simulink model "RADTRANS001"  (R2020b)
settings: Solver=VariableStepAuto  StartTime=0.0  StopTime=10.0  RelTol=1e-3
undefined symbols (not defined in the file): Line_110_C, Line_110_L, Line_110_R, Line_220_C, Line_220_L, Line_220_R, Line_35_C, Line_35_L, Line_35_R, Line_6_L, Line_6_R, Sys_f_Hz, Sys_V_net_kV, Tr_110_35_L_pu, Tr_110_35_R_pu, Tr_110_35_Sn_VA, Tr_110_35_V_HV_kV, Tr_110_35_V_LV_kV, Tr_110_6_L_pu, Tr_110_6_R_pu, Tr_110_6_Sn_VA, Tr_110_6_V_HV_kV, Tr_110_6_V_LV_kV, Tr_220_110_L_pu, Tr_220_110_R_pu, Tr_220_110_Sn_VA, Tr_220_110_V_HV_kV, Tr_220_110_V_LV_kV, Tr_35_04_L_pu, Tr_35_04_R_pu, Tr_35_04_Sn_VA, Tr_35_04_V_HV_kV, Tr_35_04_V_LV_kV, Tr_6_04_L_pu, Tr_6_04_R_pu, Tr_6_04_Sn_VA, Tr_6_04_V_HV_kV, Tr_6_04_V_LV_kV, Ts_powergui
libraries: dspstat3 x240, powerlib x169, powerlib_meascontrol x60
(part 5 of 6)

== system RADTRANS001/M_OUT_Город_2_1 ==
  Iptg_18 : Display
      settings: Format=bank
  PQptg_18 : Scope  NumInputPorts=2
  "Power0 (3ph, Instantaneous)" : powerlib_meascontrol/Measurements/Power (3ph, Instantaneous)
  Pptg_18 : Display
      settings: Format=bank
  Qptg_18 : Display
      settings: Format=bank
  RMS18 : dspstat3/RMS  run=off  directionMode=Each column  dimension=1  InputProcessing=Columns as channels (frame based)  reset_popup=None
  RMS3 : dspstat3/RMS  run=off  directionMode=Each column  dimension=1  InputProcessing=Columns as channels (frame based)  reset_popup=None
  RMS4 : dspstat3/RMS  run=off  directionMode=Each column  dimension=1  InputProcessing=Columns as channels (frame based)  reset_popup=None
  RMSpt_18 : dspstat3/RMS  run=off  directionMode=Each column  dimension=1  InputProcessing=Columns as channels (frame based)  reset_popup=None
  Real-Ima to Complex : RealImagToComplex
  S : Abs
  SSptg_18 : Scope
  Sptg_18 : Display
      settings: Format=bank
  Three-Phase V-I Measurementpt_18 : powerlib/Measurements/Three-Phase V-I Measurement  VoltageMeasurement=phase-to-ground  SetLabelV=off  LabelV=Vabc  Vpu=off  VpuLL=off  CurrentMeasurement=yes  SetLabelI=off  LabelI=Iabc  Ipu=off  Pbase=100e6  Vbase=500e3  OutputType=Complex  PhasorSimulation=off  PSBequivalent=0
  UIptg_18 : Scope  NumInputPorts=2
  Uptg_18 : Display
      settings: Format=bank
  a : PMIOPort  Side=Right
  b : PMIOPort  Port=2  Side=Right
  c : PMIOPort  Port=3  Side=Right
  A : PMIOPort  Port=4  Side=Left
  B : PMIOPort  Port=5  Side=Left
  C : PMIOPort  Port=6  Side=Left
  tag scope: I_ptg_18=global, P_ptg_18=global, Q_ptg_18=global, S_ptg_18=global, U_ptg_18=global
  wires:
  S/1 -> [S_ptg_18]
  Real-Ima to Complex/1 -> S/1
  [S_ptg_18] -> Sptg_18/1
  [S_ptg_18] -> SSptg_18/1
  [P_ptg_18] -> RMSpt_18/1
  RMSpt_18/1 -> Pptg_18/1
  RMS18/1 -> Qptg_18/1
  [U_ptg_18] -> RMS3/1
  RMS3/1 -> Uptg_18/1
  [P_ptg_18] -> Real-Ima to Complex/1
  [Q_ptg_18] -> RMS18/1
  [I_ptg_18] -> RMS4/1
  RMS4/1 -> Iptg_18/1
  [U_ptg_18] -> UIptg_18/1  "U"
  [P_ptg_18] -> PQptg_18/1  "P"
  [I_ptg_18] -> UIptg_18/2  "I"
  Three-Phase V-I Measurementpt_18/1 -> [U_ptg_18]
  [Q_ptg_18] -> Real-Ima to Complex/2
  Three-Phase V-I Measurementpt_18/2 -> [I_ptg_18]
  [U_ptg_18] -> "Power0 (3ph, Instantaneous)"/1
  [I_ptg_18] -> "Power0 (3ph, Instantaneous)"/2
  "Power0 (3ph, Instantaneous)"/2 -> [Q_ptg_18]
  "Power0 (3ph, Instantaneous)"/1 -> [P_ptg_18]
  [Q_ptg_18] -> PQptg_18/2  "Q"
  connections:
  Three-Phase V-I Measurementpt_18/LConn1 -- A/RConn1
  Three-Phase V-I Measurementpt_18/RConn1 -- a/RConn1
  Three-Phase V-I Measurementpt_18/LConn2 -- B/RConn1
  Three-Phase V-I Measurementpt_18/LConn3 -- C/RConn1
  Three-Phase V-I Measurementpt_18/RConn3 -- c/RConn1
  Three-Phase V-I Measurementpt_18/RConn2 -- b/RConn1

== system RADTRANS001/M_OUT_Город_2_2 ==
  Iptg_20 : Display
      settings: Format=bank
  PQptg_20 : Scope  NumInputPorts=2
  "Power0 (3ph, Instantaneous)" : powerlib_meascontrol/Measurements/Power (3ph, Instantaneous)
  Pptg_20 : Display
      settings: Format=bank
  Qptg_20 : Display
      settings: Format=bank
  RMS20 : dspstat3/RMS  run=off  directionMode=Each column  dimension=1  InputProcessing=Columns as channels (frame based)  reset_popup=None
  RMS3 : dspstat3/RMS  run=off  directionMode=Each column  dimension=1  InputProcessing=Columns as channels (frame based)  reset_popup=None
  RMS4 : dspstat3/RMS  run=off  directionMode=Each column  dimension=1  InputProcessing=Columns as channels (frame based)  reset_popup=None
  RMSpt_20 : dspstat3/RMS  run=off  directionMode=Each column  dimension=1  InputProcessing=Columns as channels (frame based)  reset_popup=None
  Real-Ima to Complex : RealImagToComplex
  S : Abs
  SSptg_20 : Scope
  Sptg_20 : Display
      settings: Format=bank
  Three-Phase V-I Measurementpt_20 : powerlib/Measurements/Three-Phase V-I Measurement  VoltageMeasurement=phase-to-ground  SetLabelV=off  LabelV=Vabc  Vpu=off  VpuLL=off  CurrentMeasurement=yes  SetLabelI=off  LabelI=Iabc  Ipu=off  Pbase=100e6  Vbase=500e3  OutputType=Complex  PhasorSimulation=off  PSBequivalent=0
  UIptg_20 : Scope  NumInputPorts=2
  Uptg_20 : Display
      settings: Format=bank
  a : PMIOPort  Side=Right
  b : PMIOPort  Port=2  Side=Right
  c : PMIOPort  Port=3  Side=Right
  A : PMIOPort  Port=4  Side=Left
  B : PMIOPort  Port=5  Side=Left
  C : PMIOPort  Port=6  Side=Left
  tag scope: I_ptg_20=global, P_ptg_20=global, Q_ptg_20=global, S_ptg_20=global, U_ptg_20=global
  wires:
  S/1 -> [S_ptg_20]
  Real-Ima to Complex/1 -> S/1
  [S_ptg_20] -> Sptg_20/1
  [S_ptg_20] -> SSptg_20/1
  [P_ptg_20] -> RMSpt_20/1
  RMSpt_20/1 -> Pptg_20/1
  RMS20/1 -> Qptg_20/1
  [U_ptg_20] -> RMS3/1
  RMS3/1 -> Uptg_20/1
  [P_ptg_20] -> Real-Ima to Complex/1
  [Q_ptg_20] -> RMS20/1
  [I_ptg_20] -> RMS4/1
  RMS4/1 -> Iptg_20/1
  [U_ptg_20] -> UIptg_20/1  "U"
  [P_ptg_20] -> PQptg_20/1  "P"
  [I_ptg_20] -> UIptg_20/2  "I"
  Three-Phase V-I Measurementpt_20/1 -> [U_ptg_20]
  [Q_ptg_20] -> Real-Ima to Complex/2
  Three-Phase V-I Measurementpt_20/2 -> [I_ptg_20]
  [U_ptg_20] -> "Power0 (3ph, Instantaneous)"/1
  [I_ptg_20] -> "Power0 (3ph, Instantaneous)"/2
  "Power0 (3ph, Instantaneous)"/2 -> [Q_ptg_20]
  "Power0 (3ph, Instantaneous)"/1 -> [P_ptg_20]
  [Q_ptg_20] -> PQptg_20/2  "Q"
  connections:
  Three-Phase V-I Measurementpt_20/LConn1 -- A/RConn1
  Three-Phase V-I Measurementpt_20/RConn1 -- a/RConn1
  Three-Phase V-I Measurementpt_20/LConn2 -- B/RConn1
  Three-Phase V-I Measurementpt_20/LConn3 -- C/RConn1
  Three-Phase V-I Measurementpt_20/RConn3 -- c/RConn1
  Three-Phase V-I Measurementpt_20/RConn2 -- b/RConn1

== system RADTRANS001/M_OUT_Город_2_3 ==
  Iptg_22 : Display
      settings: Format=bank
  PQptg_22 : Scope  NumInputPorts=2
  "Power0 (3ph, Instantaneous)" : powerlib_meascontrol/Measurements/Power (3ph, Instantaneous)
  Pptg_22 : Display
      settings: Format=bank
  Qptg_22 : Display
      settings: Format=bank
  RMS22 : dspstat3/RMS  run=off  directionMode=Each column  dimension=1  InputProcessing=Columns as channels (frame based)  reset_popup=None
  RMS3 : dspstat3/RMS  run=off  directionMode=Each column  dimension=1  InputProcessing=Columns as channels (frame based)  reset_popup=None
  RMS4 : dspstat3/RMS  run=off  directionMode=Each column  dimension=1  InputProcessing=Columns as channels (frame based)  reset_popup=None
  RMSpt_22 : dspstat3/RMS  run=off  directionMode=Each column  dimension=1  InputProcessing=Columns as channels (frame based)  reset_popup=None
  Real-Ima to Complex : RealImagToComplex
  S : Abs
  SSptg_22 : Scope
  Sptg_22 : Display
      settings: Format=bank
  Three-Phase V-I Measurementpt_22 : powerlib/Measurements/Three-Phase V-I Measurement  VoltageMeasurement=phase-to-ground  SetLabelV=off  LabelV=Vabc  Vpu=off  VpuLL=off  CurrentMeasurement=yes  SetLabelI=off  LabelI=Iabc  Ipu=off  Pbase=100e6  Vbase=500e3  OutputType=Complex  PhasorSimulation=off  PSBequivalent=0
  UIptg_22 : Scope  NumInputPorts=2
  Uptg_22 : Display
      settings: Format=bank
  a : PMIOPort  Side=Right
  b : PMIOPort  Port=2  Side=Right
  c : PMIOPort  Port=3  Side=Right
  A : PMIOPort  Port=4  Side=Left
  B : PMIOPort  Port=5  Side=Left
  C : PMIOPort  Port=6  Side=Left
  tag scope: I_ptg_22=global, P_ptg_22=global, Q_ptg_22=global, S_ptg_22=global, U_ptg_22=global
  wires:
  S/1 -> [S_ptg_22]
  Real-Ima to Complex/1 -> S/1
  [S_ptg_22] -> Sptg_22/1
  [S_ptg_22] -> SSptg_22/1
  [P_ptg_22] -> RMSpt_22/1
  RMSpt_22/1 -> Pptg_22/1
  RMS22/1 -> Qptg_22/1
  [U_ptg_22] -> RMS3/1
  RMS3/1 -> Uptg_22/1
  [P_ptg_22] -> Real-Ima to Complex/1
  [Q_ptg_22] -> RMS22/1
  [I_ptg_22] -> RMS4/1
  RMS4/1 -> Iptg_22/1
  [U_ptg_22] -> UIptg_22/1  "U"
  [P_ptg_22] -> PQptg_22/1  "P"
  [I_ptg_22] -> UIptg_22/2  "I"
  Three-Phase V-I Measurementpt_22/1 -> [U_ptg_22]
  [Q_ptg_22] -> Real-Ima to Complex/2
  Three-Phase V-I Measurementpt_22/2 -> [I_ptg_22]
  [U_ptg_22] -> "Power0 (3ph, Instantaneous)"/1
  [I_ptg_22] -> "Power0 (3ph, Instantaneous)"/2
  "Power0 (3ph, Instantaneous)"/2 -> [Q_ptg_22]
  "Power0 (3ph, Instantaneous)"/1 -> [P_ptg_22]
  [Q_ptg_22] -> PQptg_22/2  "Q"
  connections:
  Three-Phase V-I Measurementpt_22/LConn1 -- A/RConn1
  Three-Phase V-I Measurementpt_22/RConn1 -- a/RConn1
  Three-Phase V-I Measurementpt_22/LConn2 -- B/RConn1
  Three-Phase V-I Measurementpt_22/LConn3 -- C/RConn1
  Three-Phase V-I Measurementpt_22/RConn3 -- c/RConn1
  Three-Phase V-I Measurementpt_22/RConn2 -- b/RConn1

== system RADTRANS001/M_OUT_Город_2_4 ==
  Iptg_24 : Display
      settings: Format=bank
  PQptg_24 : Scope  NumInputPorts=2
  "Power0 (3ph, Instantaneous)" : powerlib_meascontrol/Measurements/Power (3ph, Instantaneous)
  Pptg_24 : Display
      settings: Format=bank
  Qptg_24 : Display
      settings: Format=bank
  RMS24 : dspstat3/RMS  run=off  directionMode=Each column  dimension=1  InputProcessing=Columns as channels (frame based)  reset_popup=None
  RMS3 : dspstat3/RMS  run=off  directionMode=Each column  dimension=1  InputProcessing=Columns as channels (frame based)  reset_popup=None
  RMS4 : dspstat3/RMS  run=off  directionMode=Each column  dimension=1  InputProcessing=Columns as channels (frame based)  reset_popup=None
  RMSpt_24 : dspstat3/RMS  run=off  directionMode=Each column  dimension=1  InputProcessing=Columns as channels (frame based)  reset_popup=None
  Real-Ima to Complex : RealImagToComplex
  S : Abs
  SSptg_24 : Scope
  Sptg_24 : Display
      settings: Format=bank
  Three-Phase V-I Measurementpt_24 : powerlib/Measurements/Three-Phase V-I Measurement  VoltageMeasurement=phase-to-ground  SetLabelV=off  LabelV=Vabc  Vpu=off  VpuLL=off  CurrentMeasurement=yes  SetLabelI=off  LabelI=Iabc  Ipu=off  Pbase=100e6  Vbase=500e3  OutputType=Complex  PhasorSimulation=off  PSBequivalent=0
  UIptg_24 : Scope  NumInputPorts=2
  Uptg_24 : Display
      settings: Format=bank
  a : PMIOPort  Side=Right
  b : PMIOPort  Port=2  Side=Right
  c : PMIOPort  Port=3  Side=Right
  A : PMIOPort  Port=4  Side=Left
  B : PMIOPort  Port=5  Side=Left
  C : PMIOPort  Port=6  Side=Left
  tag scope: I_ptg_24=global, P_ptg_24=global, Q_ptg_24=global, S_ptg_24=global, U_ptg_24=global
  wires:
  S/1 -> [S_ptg_24]
  Real-Ima to Complex/1 -> S/1
  [S_ptg_24] -> Sptg_24/1
  [S_ptg_24] -> SSptg_24/1
  [P_ptg_24] -> RMSpt_24/1
  RMSpt_24/1 -> Pptg_24/1
  RMS24/1 -> Qptg_24/1
  [U_ptg_24] -> RMS3/1
  RMS3/1 -> Uptg_24/1
  [P_ptg_24] -> Real-Ima to Complex/1
  [Q_ptg_24] -> RMS24/1
  [I_ptg_24] -> RMS4/1
  RMS4/1 -> Iptg_24/1
  [U_ptg_24] -> UIptg_24/1  "U"
  [P_ptg_24] -> PQptg_24/1  "P"
  [I_ptg_24] -> UIptg_24/2  "I"
  Three-Phase V-I Measurementpt_24/1 -> [U_ptg_24]
  [Q_ptg_24] -> Real-Ima to Complex/2
  Three-Phase V-I Measurementpt_24/2 -> [I_ptg_24]
  [U_ptg_24] -> "Power0 (3ph, Instantaneous)"/1
  [I_ptg_24] -> "Power0 (3ph, Instantaneous)"/2
  "Power0 (3ph, Instantaneous)"/2 -> [Q_ptg_24]
  "Power0 (3ph, Instantaneous)"/1 -> [P_ptg_24]
  [Q_ptg_24] -> PQptg_24/2  "Q"
  connections:
  Three-Phase V-I Measurementpt_24/LConn1 -- A/RConn1
  Three-Phase V-I Measurementpt_24/RConn1 -- a/RConn1
  Three-Phase V-I Measurementpt_24/LConn2 -- B/RConn1
  Three-Phase V-I Measurementpt_24/LConn3 -- C/RConn1
  Three-Phase V-I Measurementpt_24/RConn3 -- c/RConn1
  Three-Phase V-I Measurementpt_24/RConn2 -- b/RConn1

== system RADTRANS001/M_OUT_Город_3_1 ==
  Iptg_30 : Display
      settings: Format=bank
  PQptg_30 : Scope  NumInputPorts=2
  "Power0 (3ph, Instantaneous)" : powerlib_meascontrol/Measurements/Power (3ph, Instantaneous)
  Pptg_30 : Display
      settings: Format=bank
  Qptg_30 : Display
      settings: Format=bank
  RMS3 : dspstat3/RMS  run=off  directionMode=Each column  dimension=1  InputProcessing=Columns as channels (frame based)  reset_popup=None
  RMS30 : dspstat3/RMS  run=off  directionMode=Each column  dimension=1  InputProcessing=Columns as channels (frame based)  reset_popup=None
  RMS4 : dspstat3/RMS  run=off  directionMode=Each column  dimension=1  InputProcessing=Columns as channels (frame based)  reset_popup=None
  RMSpt_30 : dspstat3/RMS  run=off  directionMode=Each column  dimension=1  InputProcessing=Columns as channels (frame based)  reset_popup=None
  Real-Ima to Complex : RealImagToComplex
  S : Abs
  SSptg_30 : Scope
  Sptg_30 : Display
      settings: Format=bank
  Three-Phase V-I Measurementpt_30 : powerlib/Measurements/Three-Phase V-I Measurement  VoltageMeasurement=phase-to-ground  SetLabelV=off  LabelV=Vabc  Vpu=off  VpuLL=off  CurrentMeasurement=yes  SetLabelI=off  LabelI=Iabc  Ipu=off  Pbase=100e6  Vbase=500e3  OutputType=Complex  PhasorSimulation=off  PSBequivalent=0
  UIptg_30 : Scope  NumInputPorts=2
  Uptg_30 : Display
      settings: Format=bank
  a : PMIOPort  Side=Right
  b : PMIOPort  Port=2  Side=Right
  c : PMIOPort  Port=3  Side=Right
  A : PMIOPort  Port=4  Side=Left
  B : PMIOPort  Port=5  Side=Left
  C : PMIOPort  Port=6  Side=Left
  tag scope: I_ptg_30=global, P_ptg_30=global, Q_ptg_30=global, S_ptg_30=global, U_ptg_30=global
  wires:
  S/1 -> [S_ptg_30]
  Real-Ima to Complex/1 -> S/1
  [S_ptg_30] -> Sptg_30/1
  [S_ptg_30] -> SSptg_30/1
  [P_ptg_30] -> RMSpt_30/1
  RMSpt_30/1 -> Pptg_30/1
  RMS30/1 -> Qptg_30/1
  [U_ptg_30] -> RMS3/1
  RMS3/1 -> Uptg_30/1
  [P_ptg_30] -> Real-Ima to Complex/1
  [Q_ptg_30] -> RMS30/1
  [I_ptg_30] -> RMS4/1
  RMS4/1 -> Iptg_30/1
  [U_ptg_30] -> UIptg_30/1  "U"
  [P_ptg_30] -> PQptg_30/1  "P"
  [I_ptg_30] -> UIptg_30/2  "I"
  Three-Phase V-I Measurementpt_30/1 -> [U_ptg_30]
  [Q_ptg_30] -> Real-Ima to Complex/2
  Three-Phase V-I Measurementpt_30/2 -> [I_ptg_30]
  [U_ptg_30] -> "Power0 (3ph, Instantaneous)"/1
  [I_ptg_30] -> "Power0 (3ph, Instantaneous)"/2
  "Power0 (3ph, Instantaneous)"/2 -> [Q_ptg_30]
  "Power0 (3ph, Instantaneous)"/1 -> [P_ptg_30]
  [Q_ptg_30] -> PQptg_30/2  "Q"
  connections:
  Three-Phase V-I Measurementpt_30/LConn1 -- A/RConn1
  Three-Phase V-I Measurementpt_30/RConn1 -- a/RConn1
  Three-Phase V-I Measurementpt_30/LConn2 -- B/RConn1
  Three-Phase V-I Measurementpt_30/LConn3 -- C/RConn1
  Three-Phase V-I Measurementpt_30/RConn3 -- c/RConn1
  Three-Phase V-I Measurementpt_30/RConn2 -- b/RConn1

== system RADTRANS001/M_OUT_Город_3_2 ==
  Iptg_32 : Display
      settings: Format=bank
  PQptg_32 : Scope  NumInputPorts=2
  "Power0 (3ph, Instantaneous)" : powerlib_meascontrol/Measurements/Power (3ph, Instantaneous)
  Pptg_32 : Display
      settings: Format=bank
  Qptg_32 : Display
      settings: Format=bank
  RMS3 : dspstat3/RMS  run=off  directionMode=Each column  dimension=1  InputProcessing=Columns as channels (frame based)  reset_popup=None
  RMS32 : dspstat3/RMS  run=off  directionMode=Each column  dimension=1  InputProcessing=Columns as channels (frame based)  reset_popup=None
  RMS4 : dspstat3/RMS  run=off  directionMode=Each column  dimension=1  InputProcessing=Columns as channels (frame based)  reset_popup=None
  RMSpt_32 : dspstat3/RMS  run=off  directionMode=Each column  dimension=1  InputProcessing=Columns as channels (frame based)  reset_popup=None
  Real-Ima to Complex : RealImagToComplex
  S : Abs
  SSptg_32 : Scope
  Sptg_32 : Display
      settings: Format=bank
  Three-Phase V-I Measurementpt_32 : powerlib/Measurements/Three-Phase V-I Measurement  VoltageMeasurement=phase-to-ground  SetLabelV=off  LabelV=Vabc  Vpu=off  VpuLL=off  CurrentMeasurement=yes  SetLabelI=off  LabelI=Iabc  Ipu=off  Pbase=100e6  Vbase=500e3  OutputType=Complex  PhasorSimulation=off  PSBequivalent=0
  UIptg_32 : Scope  NumInputPorts=2
  Uptg_32 : Display
      settings: Format=bank
  a : PMIOPort  Side=Right
  b : PMIOPort  Port=2  Side=Right
  c : PMIOPort  Port=3  Side=Right
  A : PMIOPort  Port=4  Side=Left
  B : PMIOPort  Port=5  Side=Left
  C : PMIOPort  Port=6  Side=Left
  tag scope: I_ptg_32=global, P_ptg_32=global, Q_ptg_32=global, S_ptg_32=global, U_ptg_32=global
  wires:
  S/1 -> [S_ptg_32]
  Real-Ima to Complex/1 -> S/1
  [S_ptg_32] -> Sptg_32/1
  [S_ptg_32] -> SSptg_32/1
  [P_ptg_32] -> RMSpt_32/1
  RMSpt_32/1 -> Pptg_32/1
  RMS32/1 -> Qptg_32/1
  [U_ptg_32] -> RMS3/1
  RMS3/1 -> Uptg_32/1
  [P_ptg_32] -> Real-Ima to Complex/1
  [Q_ptg_32] -> RMS32/1
  [I_ptg_32] -> RMS4/1
  RMS4/1 -> Iptg_32/1
  [U_ptg_32] -> UIptg_32/1  "U"
  [P_ptg_32] -> PQptg_32/1  "P"
  [I_ptg_32] -> UIptg_32/2  "I"
  Three-Phase V-I Measurementpt_32/1 -> [U_ptg_32]
  [Q_ptg_32] -> Real-Ima to Complex/2
  Three-Phase V-I Measurementpt_32/2 -> [I_ptg_32]
  [U_ptg_32] -> "Power0 (3ph, Instantaneous)"/1
  [I_ptg_32] -> "Power0 (3ph, Instantaneous)"/2
  "Power0 (3ph, Instantaneous)"/2 -> [Q_ptg_32]
  "Power0 (3ph, Instantaneous)"/1 -> [P_ptg_32]
  [Q_ptg_32] -> PQptg_32/2  "Q"
  connections:
  Three-Phase V-I Measurementpt_32/LConn1 -- A/RConn1
  Three-Phase V-I Measurementpt_32/RConn1 -- a/RConn1
  Three-Phase V-I Measurementpt_32/LConn2 -- B/RConn1
  Three-Phase V-I Measurementpt_32/LConn3 -- C/RConn1
  Three-Phase V-I Measurementpt_32/RConn3 -- c/RConn1
  Three-Phase V-I Measurementpt_32/RConn2 -- b/RConn1

== system RADTRANS001/M_OUT_Город_3_3 ==
  Iptg_34 : Display
      settings: Format=bank
  PQptg_34 : Scope  NumInputPorts=2
  "Power0 (3ph, Instantaneous)" : powerlib_meascontrol/Measurements/Power (3ph, Instantaneous)
  Pptg_34 : Display
      settings: Format=bank
  Qptg_34 : Display
      settings: Format=bank
  RMS3 : dspstat3/RMS  run=off  directionMode=Each column  dimension=1  InputProcessing=Columns as channels (frame based)  reset_popup=None
  RMS34 : dspstat3/RMS  run=off  directionMode=Each column  dimension=1  InputProcessing=Columns as channels (frame based)  reset_popup=None
  RMS4 : dspstat3/RMS  run=off  directionMode=Each column  dimension=1  InputProcessing=Columns as channels (frame based)  reset_popup=None
  RMSpt_34 : dspstat3/RMS  run=off  directionMode=Each column  dimension=1  InputProcessing=Columns as channels (frame based)  reset_popup=None
  Real-Ima to Complex : RealImagToComplex
  S : Abs
  SSptg_34 : Scope
  Sptg_34 : Display
      settings: Format=bank
  Three-Phase V-I Measurementpt_34 : powerlib/Measurements/Three-Phase V-I Measurement  VoltageMeasurement=phase-to-ground  SetLabelV=off  LabelV=Vabc  Vpu=off  VpuLL=off  CurrentMeasurement=yes  SetLabelI=off  LabelI=Iabc  Ipu=off  Pbase=100e6  Vbase=500e3  OutputType=Complex  PhasorSimulation=off  PSBequivalent=0
  UIptg_34 : Scope  NumInputPorts=2
  Uptg_34 : Display
      settings: Format=bank
  a : PMIOPort  Side=Right
  b : PMIOPort  Port=2  Side=Right
  c : PMIOPort  Port=3  Side=Right
  A : PMIOPort  Port=4  Side=Left
  B : PMIOPort  Port=5  Side=Left
  C : PMIOPort  Port=6  Side=Left
  tag scope: I_ptg_34=global, P_ptg_34=global, Q_ptg_34=global, S_ptg_34=global, U_ptg_34=global
  wires:
  S/1 -> [S_ptg_34]
  Real-Ima to Complex/1 -> S/1
  [S_ptg_34] -> Sptg_34/1
  [S_ptg_34] -> SSptg_34/1
  [P_ptg_34] -> RMSpt_34/1
  RMSpt_34/1 -> Pptg_34/1
  RMS34/1 -> Qptg_34/1
  [U_ptg_34] -> RMS3/1
  RMS3/1 -> Uptg_34/1
  [P_ptg_34] -> Real-Ima to Complex/1
  [Q_ptg_34] -> RMS34/1
  [I_ptg_34] -> RMS4/1
  RMS4/1 -> Iptg_34/1
  [U_ptg_34] -> UIptg_34/1  "U"
  [P_ptg_34] -> PQptg_34/1  "P"
  [I_ptg_34] -> UIptg_34/2  "I"
  Three-Phase V-I Measurementpt_34/1 -> [U_ptg_34]
  [Q_ptg_34] -> Real-Ima to Complex/2
  Three-Phase V-I Measurementpt_34/2 -> [I_ptg_34]
  [U_ptg_34] -> "Power0 (3ph, Instantaneous)"/1
  [I_ptg_34] -> "Power0 (3ph, Instantaneous)"/2
  "Power0 (3ph, Instantaneous)"/2 -> [Q_ptg_34]
  "Power0 (3ph, Instantaneous)"/1 -> [P_ptg_34]
  [Q_ptg_34] -> PQptg_34/2  "Q"
  connections:
  Three-Phase V-I Measurementpt_34/LConn1 -- A/RConn1
  Three-Phase V-I Measurementpt_34/RConn1 -- a/RConn1
  Three-Phase V-I Measurementpt_34/LConn2 -- B/RConn1
  Three-Phase V-I Measurementpt_34/LConn3 -- C/RConn1
  Three-Phase V-I Measurementpt_34/RConn3 -- c/RConn1
  Three-Phase V-I Measurementpt_34/RConn2 -- b/RConn1

== system RADTRANS001/M_OUT_Город_3_4 ==
  Iptg_36 : Display
      settings: Format=bank
  PQptg_36 : Scope  NumInputPorts=2
  "Power0 (3ph, Instantaneous)" : powerlib_meascontrol/Measurements/Power (3ph, Instantaneous)
  Pptg_36 : Display
      settings: Format=bank
  Qptg_36 : Display
      settings: Format=bank
  RMS3 : dspstat3/RMS  run=off  directionMode=Each column  dimension=1  InputProcessing=Columns as channels (frame based)  reset_popup=None
  RMS36 : dspstat3/RMS  run=off  directionMode=Each column  dimension=1  InputProcessing=Columns as channels (frame based)  reset_popup=None
  RMS4 : dspstat3/RMS  run=off  directionMode=Each column  dimension=1  InputProcessing=Columns as channels (frame based)  reset_popup=None
  RMSpt_36 : dspstat3/RMS  run=off  directionMode=Each column  dimension=1  InputProcessing=Columns as channels (frame based)  reset_popup=None
  Real-Ima to Complex : RealImagToComplex
  S : Abs
  SSptg_36 : Scope
  Sptg_36 : Display
      settings: Format=bank
  Three-Phase V-I Measurementpt_36 : powerlib/Measurements/Three-Phase V-I Measurement  VoltageMeasurement=phase-to-ground  SetLabelV=off  LabelV=Vabc  Vpu=off  VpuLL=off  CurrentMeasurement=yes  SetLabelI=off  LabelI=Iabc  Ipu=off  Pbase=100e6  Vbase=500e3  OutputType=Complex  PhasorSimulation=off  PSBequivalent=0
  UIptg_36 : Scope  NumInputPorts=2
  Uptg_36 : Display
      settings: Format=bank
  a : PMIOPort  Side=Right
  b : PMIOPort  Port=2  Side=Right
  c : PMIOPort  Port=3  Side=Right
  A : PMIOPort  Port=4  Side=Left
  B : PMIOPort  Port=5  Side=Left
  C : PMIOPort  Port=6  Side=Left
  tag scope: I_ptg_36=global, P_ptg_36=global, Q_ptg_36=global, S_ptg_36=global, U_ptg_36=global
  wires:
  S/1 -> [S_ptg_36]
  Real-Ima to Complex/1 -> S/1
  [S_ptg_36] -> Sptg_36/1
  [S_ptg_36] -> SSptg_36/1
  [P_ptg_36] -> RMSpt_36/1
  RMSpt_36/1 -> Pptg_36/1
  RMS36/1 -> Qptg_36/1
  [U_ptg_36] -> RMS3/1
  RMS3/1 -> Uptg_36/1
  [P_ptg_36] -> Real-Ima to Complex/1
  [Q_ptg_36] -> RMS36/1
  [I_ptg_36] -> RMS4/1
  RMS4/1 -> Iptg_36/1
  [U_ptg_36] -> UIptg_36/1  "U"
  [P_ptg_36] -> PQptg_36/1  "P"
  [I_ptg_36] -> UIptg_36/2  "I"
  Three-Phase V-I Measurementpt_36/1 -> [U_ptg_36]
  [Q_ptg_36] -> Real-Ima to Complex/2
  Three-Phase V-I Measurementpt_36/2 -> [I_ptg_36]
  [U_ptg_36] -> "Power0 (3ph, Instantaneous)"/1
  [I_ptg_36] -> "Power0 (3ph, Instantaneous)"/2
  "Power0 (3ph, Instantaneous)"/2 -> [Q_ptg_36]
  "Power0 (3ph, Instantaneous)"/1 -> [P_ptg_36]
  [Q_ptg_36] -> PQptg_36/2  "Q"
  connections:
  Three-Phase V-I Measurementpt_36/LConn1 -- A/RConn1
  Three-Phase V-I Measurementpt_36/RConn1 -- a/RConn1
  Three-Phase V-I Measurementpt_36/LConn2 -- B/RConn1
  Three-Phase V-I Measurementpt_36/LConn3 -- C/RConn1
  Three-Phase V-I Measurementpt_36/RConn3 -- c/RConn1
  Three-Phase V-I Measurementpt_36/RConn2 -- b/RConn1

== system RADTRANS001/M_OUT_Город_4_1 ==
  Iptg_42 : Display
      settings: Format=bank
  PQptg_42 : Scope  NumInputPorts=2
  "Power0 (3ph, Instantaneous)" : powerlib_meascontrol/Measurements/Power (3ph, Instantaneous)
  Pptg_42 : Display
      settings: Format=bank
  Qptg_42 : Display
      settings: Format=bank
  RMS3 : dspstat3/RMS  run=off  directionMode=Each column  dimension=1  InputProcessing=Columns as channels (frame based)  reset_popup=None
  RMS4 : dspstat3/RMS  run=off  directionMode=Each column  dimension=1  InputProcessing=Columns as channels (frame based)  reset_popup=None
  RMS42 : dspstat3/RMS  run=off  directionMode=Each column  dimension=1  InputProcessing=Columns as channels (frame based)  reset_popup=None
  RMSpt_42 : dspstat3/RMS  run=off  directionMode=Each column  dimension=1  InputProcessing=Columns as channels (frame based)  reset_popup=None
  Real-Ima to Complex : RealImagToComplex
  S : Abs
  SSptg_42 : Scope
  Sptg_42 : Display
      settings: Format=bank
  Three-Phase V-I Measurementpt_42 : powerlib/Measurements/Three-Phase V-I Measurement  VoltageMeasurement=phase-to-ground  SetLabelV=off  LabelV=Vabc  Vpu=off  VpuLL=off  CurrentMeasurement=yes  SetLabelI=off  LabelI=Iabc  Ipu=off  Pbase=100e6  Vbase=500e3  OutputType=Complex  PhasorSimulation=off  PSBequivalent=0
  UIptg_42 : Scope  NumInputPorts=2
  Uptg_42 : Display
      settings: Format=bank
  a : PMIOPort  Side=Right
  b : PMIOPort  Port=2  Side=Right
  c : PMIOPort  Port=3  Side=Right
  A : PMIOPort  Port=4  Side=Left
  B : PMIOPort  Port=5  Side=Left
  C : PMIOPort  Port=6  Side=Left
  tag scope: I_ptg_42=global, P_ptg_42=global, Q_ptg_42=global, S_ptg_42=global, U_ptg_42=global
  wires:
  S/1 -> [S_ptg_42]
  Real-Ima to Complex/1 -> S/1
  [S_ptg_42] -> Sptg_42/1
  [S_ptg_42] -> SSptg_42/1
  [P_ptg_42] -> RMSpt_42/1
  RMSpt_42/1 -> Pptg_42/1
  RMS42/1 -> Qptg_42/1
  [U_ptg_42] -> RMS3/1
  RMS3/1 -> Uptg_42/1
  [P_ptg_42] -> Real-Ima to Complex/1
  [Q_ptg_42] -> RMS42/1
  [I_ptg_42] -> RMS4/1
  RMS4/1 -> Iptg_42/1
  [U_ptg_42] -> UIptg_42/1  "U"
  [P_ptg_42] -> PQptg_42/1  "P"
  [I_ptg_42] -> UIptg_42/2  "I"
  Three-Phase V-I Measurementpt_42/1 -> [U_ptg_42]
  [Q_ptg_42] -> Real-Ima to Complex/2
  Three-Phase V-I Measurementpt_42/2 -> [I_ptg_42]
  [U_ptg_42] -> "Power0 (3ph, Instantaneous)"/1
  [I_ptg_42] -> "Power0 (3ph, Instantaneous)"/2
  "Power0 (3ph, Instantaneous)"/2 -> [Q_ptg_42]
  "Power0 (3ph, Instantaneous)"/1 -> [P_ptg_42]
  [Q_ptg_42] -> PQptg_42/2  "Q"
  connections:
  Three-Phase V-I Measurementpt_42/LConn1 -- A/RConn1
  Three-Phase V-I Measurementpt_42/RConn1 -- a/RConn1
  Three-Phase V-I Measurementpt_42/LConn2 -- B/RConn1
  Three-Phase V-I Measurementpt_42/LConn3 -- C/RConn1
  Three-Phase V-I Measurementpt_42/RConn3 -- c/RConn1
  Three-Phase V-I Measurementpt_42/RConn2 -- b/RConn1

== system RADTRANS001/M_OUT_Город_4_2 ==
  Iptg_44 : Display
      settings: Format=bank
  PQptg_44 : Scope  NumInputPorts=2
  "Power0 (3ph, Instantaneous)" : powerlib_meascontrol/Measurements/Power (3ph, Instantaneous)
  Pptg_44 : Display
      settings: Format=bank
  Qptg_44 : Display
      settings: Format=bank
  RMS3 : dspstat3/RMS  run=off  directionMode=Each column  dimension=1  InputProcessing=Columns as channels (frame based)  reset_popup=None
  RMS4 : dspstat3/RMS  run=off  directionMode=Each column  dimension=1  InputProcessing=Columns as channels (frame based)  reset_popup=None
  RMS44 : dspstat3/RMS  run=off  directionMode=Each column  dimension=1  InputProcessing=Columns as channels (frame based)  reset_popup=None
  RMSpt_44 : dspstat3/RMS  run=off  directionMode=Each column  dimension=1  InputProcessing=Columns as channels (frame based)  reset_popup=None
  Real-Ima to Complex : RealImagToComplex
  S : Abs
  SSptg_44 : Scope
  Sptg_44 : Display
      settings: Format=bank
  Three-Phase V-I Measurementpt_44 : powerlib/Measurements/Three-Phase V-I Measurement  VoltageMeasurement=phase-to-ground  SetLabelV=off  LabelV=Vabc  Vpu=off  VpuLL=off  CurrentMeasurement=yes  SetLabelI=off  LabelI=Iabc  Ipu=off  Pbase=100e6  Vbase=500e3  OutputType=Complex  PhasorSimulation=off  PSBequivalent=0
  UIptg_44 : Scope  NumInputPorts=2
  Uptg_44 : Display
      settings: Format=bank
  a : PMIOPort  Side=Right
  b : PMIOPort  Port=2  Side=Right
  c : PMIOPort  Port=3  Side=Right
  A : PMIOPort  Port=4  Side=Left
  B : PMIOPort  Port=5  Side=Left
  C : PMIOPort  Port=6  Side=Left
  tag scope: I_ptg_44=global, P_ptg_44=global, Q_ptg_44=global, S_ptg_44=global, U_ptg_44=global
  wires:
  S/1 -> [S_ptg_44]
  Real-Ima to Complex/1 -> S/1
  [S_ptg_44] -> Sptg_44/1
  [S_ptg_44] -> SSptg_44/1
  [P_ptg_44] -> RMSpt_44/1
  RMSpt_44/1 -> Pptg_44/1
  RMS44/1 -> Qptg_44/1
  [U_ptg_44] -> RMS3/1
  RMS3/1 -> Uptg_44/1
  [P_ptg_44] -> Real-Ima to Complex/1
  [Q_ptg_44] -> RMS44/1
  [I_ptg_44] -> RMS4/1
  RMS4/1 -> Iptg_44/1
  [U_ptg_44] -> UIptg_44/1  "U"
  [P_ptg_44] -> PQptg_44/1  "P"
  [I_ptg_44] -> UIptg_44/2  "I"
  Three-Phase V-I Measurementpt_44/1 -> [U_ptg_44]
  [Q_ptg_44] -> Real-Ima to Complex/2
  Three-Phase V-I Measurementpt_44/2 -> [I_ptg_44]
  [U_ptg_44] -> "Power0 (3ph, Instantaneous)"/1
  [I_ptg_44] -> "Power0 (3ph, Instantaneous)"/2
  "Power0 (3ph, Instantaneous)"/2 -> [Q_ptg_44]
  "Power0 (3ph, Instantaneous)"/1 -> [P_ptg_44]
  [Q_ptg_44] -> PQptg_44/2  "Q"
  connections:
  Three-Phase V-I Measurementpt_44/LConn1 -- A/RConn1
  Three-Phase V-I Measurementpt_44/RConn1 -- a/RConn1
  Three-Phase V-I Measurementpt_44/LConn2 -- B/RConn1
  Three-Phase V-I Measurementpt_44/LConn3 -- C/RConn1
  Three-Phase V-I Measurementpt_44/RConn3 -- c/RConn1
  Three-Phase V-I Measurementpt_44/RConn2 -- b/RConn1

== system RADTRANS001/M_OUT_Город_4_3 ==
  Iptg_46 : Display
      settings: Format=bank
  PQptg_46 : Scope  NumInputPorts=2
  "Power0 (3ph, Instantaneous)" : powerlib_meascontrol/Measurements/Power (3ph, Instantaneous)
  Pptg_46 : Display
      settings: Format=bank
  Qptg_46 : Display
      settings: Format=bank
  RMS3 : dspstat3/RMS  run=off  directionMode=Each column  dimension=1  InputProcessing=Columns as channels (frame based)  reset_popup=None
  RMS4 : dspstat3/RMS  run=off  directionMode=Each column  dimension=1  InputProcessing=Columns as channels (frame based)  reset_popup=None
  RMS46 : dspstat3/RMS  run=off  directionMode=Each column  dimension=1  InputProcessing=Columns as channels (frame based)  reset_popup=None
  RMSpt_46 : dspstat3/RMS  run=off  directionMode=Each column  dimension=1  InputProcessing=Columns as channels (frame based)  reset_popup=None
  Real-Ima to Complex : RealImagToComplex
  S : Abs
  SSptg_46 : Scope
  Sptg_46 : Display
      settings: Format=bank
  Three-Phase V-I Measurementpt_46 : powerlib/Measurements/Three-Phase V-I Measurement  VoltageMeasurement=phase-to-ground  SetLabelV=off  LabelV=Vabc  Vpu=off  VpuLL=off  CurrentMeasurement=yes  SetLabelI=off  LabelI=Iabc  Ipu=off  Pbase=100e6  Vbase=500e3  OutputType=Complex  PhasorSimulation=off  PSBequivalent=0
  UIptg_46 : Scope  NumInputPorts=2
  Uptg_46 : Display
      settings: Format=bank
  a : PMIOPort  Side=Right
  b : PMIOPort  Port=2  Side=Right
  c : PMIOPort  Port=3  Side=Right
  A : PMIOPort  Port=4  Side=Left
  B : PMIOPort  Port=5  Side=Left
  C : PMIOPort  Port=6  Side=Left
  tag scope: I_ptg_46=global, P_ptg_46=global, Q_ptg_46=global, S_ptg_46=global, U_ptg_46=global
  wires:
  S/1 -> [S_ptg_46]
  Real-Ima to Complex/1 -> S/1
  [S_ptg_46] -> Sptg_46/1
  [S_ptg_46] -> SSptg_46/1
  [P_ptg_46] -> RMSpt_46/1
  RMSpt_46/1 -> Pptg_46/1
  RMS46/1 -> Qptg_46/1
  [U_ptg_46] -> RMS3/1
  RMS3/1 -> Uptg_46/1
  [P_ptg_46] -> Real-Ima to Complex/1
  [Q_ptg_46] -> RMS46/1
  [I_ptg_46] -> RMS4/1
  RMS4/1 -> Iptg_46/1
  [U_ptg_46] -> UIptg_46/1  "U"
  [P_ptg_46] -> PQptg_46/1  "P"
  [I_ptg_46] -> UIptg_46/2  "I"
  Three-Phase V-I Measurementpt_46/1 -> [U_ptg_46]
  [Q_ptg_46] -> Real-Ima to Complex/2
  Three-Phase V-I Measurementpt_46/2 -> [I_ptg_46]
  [U_ptg_46] -> "Power0 (3ph, Instantaneous)"/1
  [I_ptg_46] -> "Power0 (3ph, Instantaneous)"/2
  "Power0 (3ph, Instantaneous)"/2 -> [Q_ptg_46]
  "Power0 (3ph, Instantaneous)"/1 -> [P_ptg_46]
  [Q_ptg_46] -> PQptg_46/2  "Q"
  connections:
  Three-Phase V-I Measurementpt_46/LConn1 -- A/RConn1
  Three-Phase V-I Measurementpt_46/RConn1 -- a/RConn1
  Three-Phase V-I Measurementpt_46/LConn2 -- B/RConn1
  Three-Phase V-I Measurementpt_46/LConn3 -- C/RConn1
  Three-Phase V-I Measurementpt_46/RConn3 -- c/RConn1
  Three-Phase V-I Measurementpt_46/RConn2 -- b/RConn1

== system RADTRANS001/M_OUT_Город_4_4 ==
  Iptg_48 : Display
      settings: Format=bank
  PQptg_48 : Scope  NumInputPorts=2
  "Power0 (3ph, Instantaneous)" : powerlib_meascontrol/Measurements/Power (3ph, Instantaneous)
  Pptg_48 : Display
      settings: Format=bank
  Qptg_48 : Display
      settings: Format=bank
  RMS3 : dspstat3/RMS  run=off  directionMode=Each column  dimension=1  InputProcessing=Columns as channels (frame based)  reset_popup=None
  RMS4 : dspstat3/RMS  run=off  directionMode=Each column  dimension=1  InputProcessing=Columns as channels (frame based)  reset_popup=None
  RMS48 : dspstat3/RMS  run=off  directionMode=Each column  dimension=1  InputProcessing=Columns as channels (frame based)  reset_popup=None
  RMSpt_48 : dspstat3/RMS  run=off  directionMode=Each column  dimension=1  InputProcessing=Columns as channels (frame based)  reset_popup=None
  Real-Ima to Complex : RealImagToComplex
  S : Abs
  SSptg_48 : Scope
  Sptg_48 : Display
      settings: Format=bank
  Three-Phase V-I Measurementpt_48 : powerlib/Measurements/Three-Phase V-I Measurement  VoltageMeasurement=phase-to-ground  SetLabelV=off  LabelV=Vabc  Vpu=off  VpuLL=off  CurrentMeasurement=yes  SetLabelI=off  LabelI=Iabc  Ipu=off  Pbase=100e6  Vbase=500e3  OutputType=Complex  PhasorSimulation=off  PSBequivalent=0
  UIptg_48 : Scope  NumInputPorts=2
  Uptg_48 : Display
      settings: Format=bank
  a : PMIOPort  Side=Right
  b : PMIOPort  Port=2  Side=Right
  c : PMIOPort  Port=3  Side=Right
  A : PMIOPort  Port=4  Side=Left
  B : PMIOPort  Port=5  Side=Left
  C : PMIOPort  Port=6  Side=Left
  tag scope: I_ptg_48=global, P_ptg_48=global, Q_ptg_48=global, S_ptg_48=global, U_ptg_48=global
  wires:
  S/1 -> [S_ptg_48]
  Real-Ima to Complex/1 -> S/1
  [S_ptg_48] -> Sptg_48/1
  [S_ptg_48] -> SSptg_48/1
  [P_ptg_48] -> RMSpt_48/1
  RMSpt_48/1 -> Pptg_48/1
  RMS48/1 -> Qptg_48/1
  [U_ptg_48] -> RMS3/1
  RMS3/1 -> Uptg_48/1
  [P_ptg_48] -> Real-Ima to Complex/1
  [Q_ptg_48] -> RMS48/1
  [I_ptg_48] -> RMS4/1
  RMS4/1 -> Iptg_48/1
  [U_ptg_48] -> UIptg_48/1  "U"
  [P_ptg_48] -> PQptg_48/1  "P"
  [I_ptg_48] -> UIptg_48/2  "I"
  Three-Phase V-I Measurementpt_48/1 -> [U_ptg_48]
  [Q_ptg_48] -> Real-Ima to Complex/2
  Three-Phase V-I Measurementpt_48/2 -> [I_ptg_48]
  [U_ptg_48] -> "Power0 (3ph, Instantaneous)"/1
  [I_ptg_48] -> "Power0 (3ph, Instantaneous)"/2
  "Power0 (3ph, Instantaneous)"/2 -> [Q_ptg_48]
  "Power0 (3ph, Instantaneous)"/1 -> [P_ptg_48]
  [Q_ptg_48] -> PQptg_48/2  "Q"
  connections:
  Three-Phase V-I Measurementpt_48/LConn1 -- A/RConn1
  Three-Phase V-I Measurementpt_48/RConn1 -- a/RConn1
  Three-Phase V-I Measurementpt_48/LConn2 -- B/RConn1
  Three-Phase V-I Measurementpt_48/LConn3 -- C/RConn1
  Three-Phase V-I Measurementpt_48/RConn3 -- c/RConn1
  Three-Phase V-I Measurementpt_48/RConn2 -- b/RConn1

== system RADTRANS001/M_OUT_Город_5_1 ==
  Iptg_54 : Display
      settings: Format=bank
  PQptg_54 : Scope  NumInputPorts=2
  "Power0 (3ph, Instantaneous)" : powerlib_meascontrol/Measurements/Power (3ph, Instantaneous)
  Pptg_54 : Display
      settings: Format=bank
  Qptg_54 : Display
      settings: Format=bank
  RMS3 : dspstat3/RMS  run=off  directionMode=Each column  dimension=1  InputProcessing=Columns as channels (frame based)  reset_popup=None
  RMS4 : dspstat3/RMS  run=off  directionMode=Each column  dimension=1  InputProcessing=Columns as channels (frame based)  reset_popup=None
  RMS54 : dspstat3/RMS  run=off  directionMode=Each column  dimension=1  InputProcessing=Columns as channels (frame based)  reset_popup=None
  RMSpt_54 : dspstat3/RMS  run=off  directionMode=Each column  dimension=1  InputProcessing=Columns as channels (frame based)  reset_popup=None
  Real-Ima to Complex : RealImagToComplex
  S : Abs
  SSptg_54 : Scope
  Sptg_54 : Display
      settings: Format=bank
  Three-Phase V-I Measurementpt_54 : powerlib/Measurements/Three-Phase V-I Measurement  VoltageMeasurement=phase-to-ground  SetLabelV=off  LabelV=Vabc  Vpu=off  VpuLL=off  CurrentMeasurement=yes  SetLabelI=off  LabelI=Iabc  Ipu=off  Pbase=100e6  Vbase=500e3  OutputType=Complex  PhasorSimulation=off  PSBequivalent=0
  UIptg_54 : Scope  NumInputPorts=2
  Uptg_54 : Display
      settings: Format=bank
  a : PMIOPort  Side=Right
  b : PMIOPort  Port=2  Side=Right
  c : PMIOPort  Port=3  Side=Right
  A : PMIOPort  Port=4  Side=Left
  B : PMIOPort  Port=5  Side=Left
  C : PMIOPort  Port=6  Side=Left
  tag scope: I_ptg_54=global, P_ptg_54=global, Q_ptg_54=global, S_ptg_54=global, U_ptg_54=global
  wires:
  S/1 -> [S_ptg_54]
  Real-Ima to Complex/1 -> S/1
  [S_ptg_54] -> Sptg_54/1
  [S_ptg_54] -> SSptg_54/1
  [P_ptg_54] -> RMSpt_54/1
  RMSpt_54/1 -> Pptg_54/1
  RMS54/1 -> Qptg_54/1
  [U_ptg_54] -> RMS3/1
  RMS3/1 -> Uptg_54/1
  [P_ptg_54] -> Real-Ima to Complex/1
  [Q_ptg_54] -> RMS54/1
  [I_ptg_54] -> RMS4/1
  RMS4/1 -> Iptg_54/1
  [U_ptg_54] -> UIptg_54/1  "U"
  [P_ptg_54] -> PQptg_54/1  "P"
  [I_ptg_54] -> UIptg_54/2  "I"
  Three-Phase V-I Measurementpt_54/1 -> [U_ptg_54]
  [Q_ptg_54] -> Real-Ima to Complex/2
  Three-Phase V-I Measurementpt_54/2 -> [I_ptg_54]
  [U_ptg_54] -> "Power0 (3ph, Instantaneous)"/1
  [I_ptg_54] -> "Power0 (3ph, Instantaneous)"/2
  "Power0 (3ph, Instantaneous)"/2 -> [Q_ptg_54]
  "Power0 (3ph, Instantaneous)"/1 -> [P_ptg_54]
  [Q_ptg_54] -> PQptg_54/2  "Q"
  connections:
  Three-Phase V-I Measurementpt_54/LConn1 -- A/RConn1
  Three-Phase V-I Measurementpt_54/RConn1 -- a/RConn1
  Three-Phase V-I Measurementpt_54/LConn2 -- B/RConn1
  Three-Phase V-I Measurementpt_54/LConn3 -- C/RConn1
  Three-Phase V-I Measurementpt_54/RConn3 -- c/RConn1
  Three-Phase V-I Measurementpt_54/RConn2 -- b/RConn1

== system RADTRANS001/M_OUT_Город_5_2 ==
  Iptg_56 : Display
      settings: Format=bank
  PQptg_56 : Scope  NumInputPorts=2
  "Power0 (3ph, Instantaneous)" : powerlib_meascontrol/Measurements/Power (3ph, Instantaneous)
  Pptg_56 : Display
      settings: Format=bank
  Qptg_56 : Display
      settings: Format=bank
  RMS3 : dspstat3/RMS  run=off  directionMode=Each column  dimension=1  InputProcessing=Columns as channels (frame based)  reset_popup=None
  RMS4 : dspstat3/RMS  run=off  directionMode=Each column  dimension=1  InputProcessing=Columns as channels (frame based)  reset_popup=None
  RMS56 : dspstat3/RMS  run=off  directionMode=Each column  dimension=1  InputProcessing=Columns as channels (frame based)  reset_popup=None
  RMSpt_56 : dspstat3/RMS  run=off  directionMode=Each column  dimension=1  InputProcessing=Columns as channels (frame based)  reset_popup=None
  Real-Ima to Complex : RealImagToComplex
  S : Abs
  SSptg_56 : Scope
  Sptg_56 : Display
      settings: Format=bank
  Three-Phase V-I Measurementpt_56 : powerlib/Measurements/Three-Phase V-I Measurement  VoltageMeasurement=phase-to-ground  SetLabelV=off  LabelV=Vabc  Vpu=off  VpuLL=off  CurrentMeasurement=yes  SetLabelI=off  LabelI=Iabc  Ipu=off  Pbase=100e6  Vbase=500e3  OutputType=Complex  PhasorSimulation=off  PSBequivalent=0
  UIptg_56 : Scope  NumInputPorts=2
  Uptg_56 : Display
      settings: Format=bank
  a : PMIOPort  Side=Right
  b : PMIOPort  Port=2  Side=Right
  c : PMIOPort  Port=3  Side=Right
  A : PMIOPort  Port=4  Side=Left
  B : PMIOPort  Port=5  Side=Left
  C : PMIOPort  Port=6  Side=Left
  tag scope: I_ptg_56=global, P_ptg_56=global, Q_ptg_56=global, S_ptg_56=global, U_ptg_56=global
  wires:
  S/1 -> [S_ptg_56]
  Real-Ima to Complex/1 -> S/1
  [S_ptg_56] -> Sptg_56/1
  [S_ptg_56] -> SSptg_56/1
  [P_ptg_56] -> RMSpt_56/1
  RMSpt_56/1 -> Pptg_56/1
  RMS56/1 -> Qptg_56/1
  [U_ptg_56] -> RMS3/1
  RMS3/1 -> Uptg_56/1
  [P_ptg_56] -> Real-Ima to Complex/1
  [Q_ptg_56] -> RMS56/1
  [I_ptg_56] -> RMS4/1
  RMS4/1 -> Iptg_56/1
  [U_ptg_56] -> UIptg_56/1  "U"
  [P_ptg_56] -> PQptg_56/1  "P"
  [I_ptg_56] -> UIptg_56/2  "I"
  Three-Phase V-I Measurementpt_56/1 -> [U_ptg_56]
  [Q_ptg_56] -> Real-Ima to Complex/2
  Three-Phase V-I Measurementpt_56/2 -> [I_ptg_56]
  [U_ptg_56] -> "Power0 (3ph, Instantaneous)"/1
  [I_ptg_56] -> "Power0 (3ph, Instantaneous)"/2
  "Power0 (3ph, Instantaneous)"/2 -> [Q_ptg_56]
  "Power0 (3ph, Instantaneous)"/1 -> [P_ptg_56]
  [Q_ptg_56] -> PQptg_56/2  "Q"
  connections:
  Three-Phase V-I Measurementpt_56/LConn1 -- A/RConn1
  Three-Phase V-I Measurementpt_56/RConn1 -- a/RConn1
  Three-Phase V-I Measurementpt_56/LConn2 -- B/RConn1
  Three-Phase V-I Measurementpt_56/LConn3 -- C/RConn1
  Three-Phase V-I Measurementpt_56/RConn3 -- c/RConn1
  Three-Phase V-I Measurementpt_56/RConn2 -- b/RConn1

== system RADTRANS001/M_OUT_Город_5_3 ==
  Iptg_58 : Display
      settings: Format=bank
  PQptg_58 : Scope  NumInputPorts=2
  "Power0 (3ph, Instantaneous)" : powerlib_meascontrol/Measurements/Power (3ph, Instantaneous)
  Pptg_58 : Display
      settings: Format=bank
  Qptg_58 : Display
      settings: Format=bank
  RMS3 : dspstat3/RMS  run=off  directionMode=Each column  dimension=1  InputProcessing=Columns as channels (frame based)  reset_popup=None
  RMS4 : dspstat3/RMS  run=off  directionMode=Each column  dimension=1  InputProcessing=Columns as channels (frame based)  reset_popup=None
  RMS58 : dspstat3/RMS  run=off  directionMode=Each column  dimension=1  InputProcessing=Columns as channels (frame based)  reset_popup=None
  RMSpt_58 : dspstat3/RMS  run=off  directionMode=Each column  dimension=1  InputProcessing=Columns as channels (frame based)  reset_popup=None
  Real-Ima to Complex : RealImagToComplex
  S : Abs
  SSptg_58 : Scope
  Sptg_58 : Display
      settings: Format=bank
  Three-Phase V-I Measurementpt_58 : powerlib/Measurements/Three-Phase V-I Measurement  VoltageMeasurement=phase-to-ground  SetLabelV=off  LabelV=Vabc  Vpu=off  VpuLL=off  CurrentMeasurement=yes  SetLabelI=off  LabelI=Iabc  Ipu=off  Pbase=100e6  Vbase=500e3  OutputType=Complex  PhasorSimulation=off  PSBequivalent=0
  UIptg_58 : Scope  NumInputPorts=2
  Uptg_58 : Display
      settings: Format=bank
  a : PMIOPort  Side=Right
  b : PMIOPort  Port=2  Side=Right
  c : PMIOPort  Port=3  Side=Right
  A : PMIOPort  Port=4  Side=Left
  B : PMIOPort  Port=5  Side=Left
  C : PMIOPort  Port=6  Side=Left
  tag scope: I_ptg_58=global, P_ptg_58=global, Q_ptg_58=global, S_ptg_58=global, U_ptg_58=global
  wires:
  S/1 -> [S_ptg_58]
  Real-Ima to Complex/1 -> S/1
  [S_ptg_58] -> Sptg_58/1
  [S_ptg_58] -> SSptg_58/1
  [P_ptg_58] -> RMSpt_58/1
  RMSpt_58/1 -> Pptg_58/1
  RMS58/1 -> Qptg_58/1
  [U_ptg_58] -> RMS3/1
  RMS3/1 -> Uptg_58/1
  [P_ptg_58] -> Real-Ima to Complex/1
  [Q_ptg_58] -> RMS58/1
  [I_ptg_58] -> RMS4/1
  RMS4/1 -> Iptg_58/1
  [U_ptg_58] -> UIptg_58/1  "U"
  [P_ptg_58] -> PQptg_58/1  "P"
  [I_ptg_58] -> UIptg_58/2  "I"
  Three-Phase V-I Measurementpt_58/1 -> [U_ptg_58]
  [Q_ptg_58] -> Real-Ima to Complex/2
  Three-Phase V-I Measurementpt_58/2 -> [I_ptg_58]
  [U_ptg_58] -> "Power0 (3ph, Instantaneous)"/1
  [I_ptg_58] -> "Power0 (3ph, Instantaneous)"/2
  "Power0 (3ph, Instantaneous)"/2 -> [Q_ptg_58]
  "Power0 (3ph, Instantaneous)"/1 -> [P_ptg_58]
  [Q_ptg_58] -> PQptg_58/2  "Q"
  connections:
  Three-Phase V-I Measurementpt_58/LConn1 -- A/RConn1
  Three-Phase V-I Measurementpt_58/RConn1 -- a/RConn1
  Three-Phase V-I Measurementpt_58/LConn2 -- B/RConn1
  Three-Phase V-I Measurementpt_58/LConn3 -- C/RConn1
  Three-Phase V-I Measurementpt_58/RConn3 -- c/RConn1
  Three-Phase V-I Measurementpt_58/RConn2 -- b/RConn1

== system RADTRANS001/M_OUT_Город_5_4 ==
  Iptg_60 : Display
      settings: Format=bank
  PQptg_60 : Scope  NumInputPorts=2
  "Power0 (3ph, Instantaneous)" : powerlib_meascontrol/Measurements/Power (3ph, Instantaneous)
  Pptg_60 : Display
      settings: Format=bank
  Qptg_60 : Display
      settings: Format=bank
  RMS3 : dspstat3/RMS  run=off  directionMode=Each column  dimension=1  InputProcessing=Columns as channels (frame based)  reset_popup=None
  RMS4 : dspstat3/RMS  run=off  directionMode=Each column  dimension=1  InputProcessing=Columns as channels (frame based)  reset_popup=None
  RMS60 : dspstat3/RMS  run=off  directionMode=Each column  dimension=1  InputProcessing=Columns as channels (frame based)  reset_popup=None
  RMSpt_60 : dspstat3/RMS  run=off  directionMode=Each column  dimension=1  InputProcessing=Columns as channels (frame based)  reset_popup=None
  Real-Ima to Complex : RealImagToComplex
  S : Abs
  SSptg_60 : Scope
  Sptg_60 : Display
      settings: Format=bank
  Three-Phase V-I Measurementpt_60 : powerlib/Measurements/Three-Phase V-I Measurement  VoltageMeasurement=phase-to-ground  SetLabelV=off  LabelV=Vabc  Vpu=off  VpuLL=off  CurrentMeasurement=yes  SetLabelI=off  LabelI=Iabc  Ipu=off  Pbase=100e6  Vbase=500e3  OutputType=Complex  PhasorSimulation=off  PSBequivalent=0
  UIptg_60 : Scope  NumInputPorts=2
  Uptg_60 : Display
      settings: Format=bank
  a : PMIOPort  Side=Right
  b : PMIOPort  Port=2  Side=Right
  c : PMIOPort  Port=3  Side=Right
  A : PMIOPort  Port=4  Side=Left
  B : PMIOPort  Port=5  Side=Left
  C : PMIOPort  Port=6  Side=Left
  tag scope: I_ptg_60=global, P_ptg_60=global, Q_ptg_60=global, S_ptg_60=global, U_ptg_60=global
  wires:
  S/1 -> [S_ptg_60]
  Real-Ima to Complex/1 -> S/1
  [S_ptg_60] -> Sptg_60/1
  [S_ptg_60] -> SSptg_60/1
  [P_ptg_60] -> RMSpt_60/1
  RMSpt_60/1 -> Pptg_60/1
  RMS60/1 -> Qptg_60/1
  [U_ptg_60] -> RMS3/1
  RMS3/1 -> Uptg_60/1
  [P_ptg_60] -> Real-Ima to Complex/1
  [Q_ptg_60] -> RMS60/1
  [I_ptg_60] -> RMS4/1
  RMS4/1 -> Iptg_60/1
  [U_ptg_60] -> UIptg_60/1  "U"
  [P_ptg_60] -> PQptg_60/1  "P"
  [I_ptg_60] -> UIptg_60/2  "I"
  Three-Phase V-I Measurementpt_60/1 -> [U_ptg_60]
  [Q_ptg_60] -> Real-Ima to Complex/2
  Three-Phase V-I Measurementpt_60/2 -> [I_ptg_60]
  [U_ptg_60] -> "Power0 (3ph, Instantaneous)"/1
  [I_ptg_60] -> "Power0 (3ph, Instantaneous)"/2
  "Power0 (3ph, Instantaneous)"/2 -> [Q_ptg_60]
  "Power0 (3ph, Instantaneous)"/1 -> [P_ptg_60]
  [Q_ptg_60] -> PQptg_60/2  "Q"
  connections:
  Three-Phase V-I Measurementpt_60/LConn1 -- A/RConn1
  Three-Phase V-I Measurementpt_60/RConn1 -- a/RConn1
  Three-Phase V-I Measurementpt_60/LConn2 -- B/RConn1
  Three-Phase V-I Measurementpt_60/LConn3 -- C/RConn1
  Three-Phase V-I Measurementpt_60/RConn3 -- c/RConn1
  Three-Phase V-I Measurementpt_60/RConn2 -- b/RConn1

== system RADTRANS001/M_OUT_Завод_1_1 ==
  Iptg_2 : Display
      settings: Format=bank
  PQptg_2 : Scope  NumInputPorts=2
  "Power0 (3ph, Instantaneous)" : powerlib_meascontrol/Measurements/Power (3ph, Instantaneous)
  Pptg_2 : Display
      settings: Format=bank
  Qptg_2 : Display
      settings: Format=bank
  RMS2 : dspstat3/RMS  run=off  directionMode=Each column  dimension=1  InputProcessing=Columns as channels (frame based)  reset_popup=None
  RMS3 : dspstat3/RMS  run=off  directionMode=Each column  dimension=1  InputProcessing=Columns as channels (frame based)  reset_popup=None
  RMS4 : dspstat3/RMS  run=off  directionMode=Each column  dimension=1  InputProcessing=Columns as channels (frame based)  reset_popup=None
  RMSpt_2 : dspstat3/RMS  run=off  directionMode=Each column  dimension=1  InputProcessing=Columns as channels (frame based)  reset_popup=None
  Real-Ima to Complex : RealImagToComplex
  S : Abs
  SSptg_2 : Scope
  Sptg_2 : Display
      settings: Format=bank
  Three-Phase V-I Measurementpt_2 : powerlib/Measurements/Three-Phase V-I Measurement  VoltageMeasurement=phase-to-ground  SetLabelV=off  LabelV=Vabc  Vpu=off  VpuLL=off  CurrentMeasurement=yes  SetLabelI=off  LabelI=Iabc  Ipu=off  Pbase=100e6  Vbase=500e3  OutputType=Complex  PhasorSimulation=off  PSBequivalent=0
  UIptg_2 : Scope  NumInputPorts=2
  Uptg_2 : Display
      settings: Format=bank
  a : PMIOPort  Side=Right
  b : PMIOPort  Port=2  Side=Right
  c : PMIOPort  Port=3  Side=Right
  A : PMIOPort  Port=4  Side=Left
  B : PMIOPort  Port=5  Side=Left
  C : PMIOPort  Port=6  Side=Left
  tag scope: I_ptg_2=global, P_ptg_2=global, Q_ptg_2=global, S_ptg_2=global, U_ptg_2=global
  wires:
  S/1 -> [S_ptg_2]
  Real-Ima to Complex/1 -> S/1
  [S_ptg_2] -> Sptg_2/1
  [S_ptg_2] -> SSptg_2/1
  [P_ptg_2] -> RMSpt_2/1
  RMSpt_2/1 -> Pptg_2/1
  RMS2/1 -> Qptg_2/1
  [U_ptg_2] -> RMS3/1
  RMS3/1 -> Uptg_2/1
  [P_ptg_2] -> Real-Ima to Complex/1
  [Q_ptg_2] -> RMS2/1
  [I_ptg_2] -> RMS4/1
  RMS4/1 -> Iptg_2/1
  [U_ptg_2] -> UIptg_2/1  "U"
  [P_ptg_2] -> PQptg_2/1  "P"
  [I_ptg_2] -> UIptg_2/2  "I"
  Three-Phase V-I Measurementpt_2/1 -> [U_ptg_2]
  [Q_ptg_2] -> Real-Ima to Complex/2
  Three-Phase V-I Measurementpt_2/2 -> [I_ptg_2]
  [U_ptg_2] -> "Power0 (3ph, Instantaneous)"/1
  [I_ptg_2] -> "Power0 (3ph, Instantaneous)"/2
  "Power0 (3ph, Instantaneous)"/2 -> [Q_ptg_2]
  "Power0 (3ph, Instantaneous)"/1 -> [P_ptg_2]
  [Q_ptg_2] -> PQptg_2/2  "Q"
  connections:
  Three-Phase V-I Measurementpt_2/LConn1 -- A/RConn1
  Three-Phase V-I Measurementpt_2/RConn1 -- a/RConn1
  Three-Phase V-I Measurementpt_2/LConn2 -- B/RConn1
  Three-Phase V-I Measurementpt_2/LConn3 -- C/RConn1
  Three-Phase V-I Measurementpt_2/RConn3 -- c/RConn1
  Three-Phase V-I Measurementpt_2/RConn2 -- b/RConn1
